simulink model "FLIGHT_Hexacopter_V2_1"  (R2024a)
settings: Solver=FixedStepDiscrete  StartTime=0.0  StopTime=inf  FixedStep=SampleTime_SAS  RelTol=1e-3  EnableMultiTasking=on
InitFcn:
  | Init_FLIGHT_Hexacopter
values from neighbouring files (symbols this model uses):
  d2r = pi/180    (= 0.0174532925199)    [Init_FLIGHT_Hexacopter.m]
  Jxx = 0.0211    [Init_FLIGHT_Hexacopter.m]
  Jyy = 0.0219    [Init_FLIGHT_Hexacopter.m]
  Jzz = 0.0366    [Init_FLIGHT_Hexacopter.m]
  Kpp = 3.3894    [Init_FLIGHT_Hexacopter_fromNCMS.m]
  Kpr = 3.3894    [Init_FLIGHT_Hexacopter_fromNCMS.m]
  MAX_CONTROL_ANGLE_PITCH = 30*pi/180    (= 0.523598775598)    [Init_FLIGHT_Hexacopter.m]    (also in Init_FLIGHT_Hexacopter_fromNCMS.m = 0.349065850399)
  MAX_CONTROL_ANGLE_RATE_PITCH = 360*pi/180    (= 6.28318530718)    [Init_FLIGHT_Hexacopter.m]    (also in Init_FLIGHT_Hexacopter_fromNCMS.m)
  MAX_CONTROL_ANGLE_RATE_ROLL = 360*pi/180    (= 6.28318530718)    [Init_FLIGHT_Hexacopter.m]    (also in Init_FLIGHT_Hexacopter_fromNCMS.m)
  MAX_CONTROL_ANGLE_RATE_Y = 120*pi/180    (= 2.09439510239)    [Init_FLIGHT_Hexacopter.m]    (also in Init_FLIGHT_Hexacopter_fromNCMS.m)
  MAX_CONTROL_ANGLE_ROLL = 30*pi/180    (= 0.523598775598)    [Init_FLIGHT_Hexacopter.m]    (also in Init_FLIGHT_Hexacopter_fromNCMS.m = 0.349065850399)
  MAX_CONTROL_VELOCITY_XY = 1.5    [Init_FLIGHT_Hexacopter.m]    (also in Init_FLIGHT_Hexacopter_fromNCMS.m)
  MAX_CONTROL_VELOCITY_Z = 1    [Init_FLIGHT_Hexacopter.m]    (also in Init_FLIGHT_Hexacopter_fromNCMS.m)
  SampleTime = 1/250    (= 0.004)    [Init_FLIGHT_Hexacopter.m]    (also in Init_FLIGHT_Hexacopter_fromNCMS.m = 0.01)
  SampleTime_SAS = 1/1000    (= 0.001)    [Init_FLIGHT_Hexacopter.m]
undefined symbols (not defined in the file or in its folder): arguments, DiscIntNeverNeededParam, event_sequence, id, log_levels, MPC_Z_D, MPC_Z_I, MPC_Z_P, timestamp
libraries: px4lib x42, simulink x9, px4Utilslib x8, px4uORBlib x8, slpidlib x5, simulink_extras x2, sharedtransform x1, px4Sensorslib x1, matrix_library x1
(part 1 of 3)
settings Model: ExtModeTrigDuration=10  Creator=sslee  LastModifiedBy=sslee
settings SolverCC: AlgebraicLoopSolver=TrustRegion  PositivePriorityOrder=on  MaxZcPerStep=1
settings OptimizationCC: EnhancedBackFolding=on  PassReuseOutputArgsAs=Individual arguments  ZeroExternalMemoryAtStartup=off  ZeroInternalMemoryAtStartup=off  MaxStackSize=64  OptimizeBlockOrder=speed  DifferentSizesBufferReuse=on  OptimizationCustomize=off  EfficientTunableParamExpr=on
settings DebuggingCC: ParameterTunabilityLossMsg=error  UnconnectedInputMsg=warning  UnconnectedOutputMsg=warning  UnconnectedLineMsg=warning  SymbolicDimsDataTypeCodeGenerationDiagnostic=none
settings HardwareCC: ProdBitPerPointer=32  ProdBitPerSizeT=32  ProdBitPerPtrDiffT=32  ProdLargestAtomicInteger=Long  ProdLargestAtomicFloat=Double  ProdWordSize=32  ProdLongLongMode=on  ProdHWDeviceType=ARM Compatible->ARM Cortex
settings ModelReferenceCC: EnableRefExpFcnMdlSchedulingChecks=on
settings SFSimCC: MATLABDynamicMemAlloc=off  SimTargetLang=C++
settings RTWCC: Description=Embedded Coder  SystemTargetFile=ert.tlc  HardwareBoard=PX4 Pixhawk 6x  TLCOptions="-aInlineSetEventsForThisBaseRateFcn=TLC_FALSE -aSuppressMultiTaskScheduler=TLC_FALSE  -aRateBasedStepFcn=0"  TemplateMakefile=ert_default_tmf  Toolchain=GNU Tools for PX4 Autopilots  IncludeHyperlinkInReport=on  TargetLang=C++  GPUComputeCapability=3.5  DLArmComputeVersion=19.05
settings CodeAppCC: ForceParamTrailComments=on  IgnoreCustomStorageClasses=off  OperatorAnnotations=on  SimulinkDataObjDesc=on  SFDataObjDesc=on  InsertBlockDesc=on
settings ERTTargetCC: ExtModeTransport=3  ExtModeStaticAlloc=on  ExtModeStaticAllocSize=1024  ExtModeMexFile=ext_xcp  ExtModeIntrfLevel=Level2 - Open

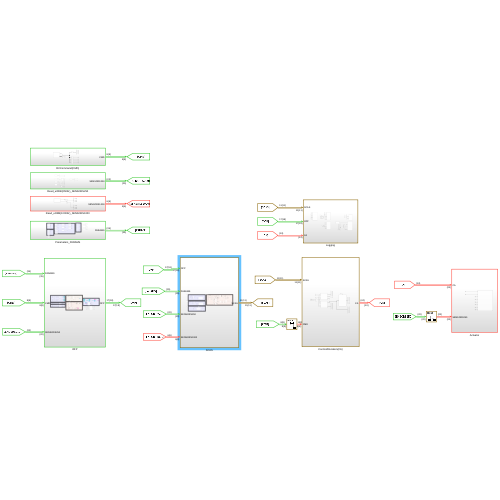
[thumbnail: Simulink's stored preview of the top-level diagram]
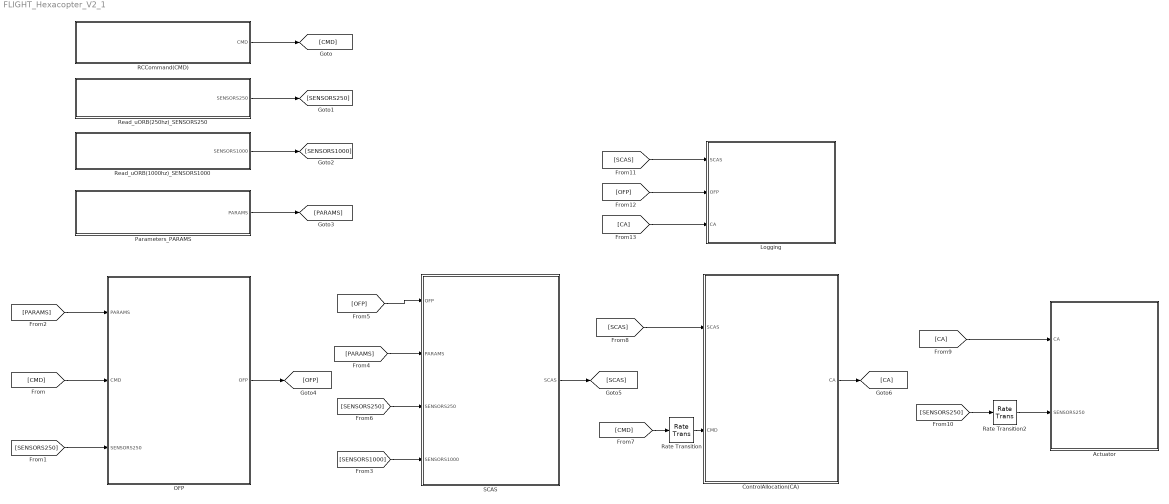
== system FLIGHT_Hexacopter_V2_1 ==
  Actuator : Subsystem
  ControlAllocation(CA) : Subsystem
  Logging : Subsystem
  OFP : Subsystem
  Parameters_PARAMS : Subsystem
  RCCommand(CMD) : Subsystem
  Rate Transition : RateTransition  OutPortSampleTime=SampleTime_SAS
  Rate Transition2 : RateTransition  OutPortSampleTime=SampleTime_SAS
  Read_uORB(1000hz)_SENSORS1000 : Subsystem
  Read_uORB(250hz)_SENSORS250 : Subsystem
  SCAS : Subsystem
  wires:
  [SENSORS250] -> OFP/3(SENSORS250)
  Read_uORB(1000hz)_SENSORS1000/1(SENSORS1000) -> [SENSORS1000]
  RCCommand(CMD)/1(CMD) -> [CMD]
  Read_uORB(250hz)_SENSORS250/1(SENSORS250) -> [SENSORS250]
  [CMD] -> OFP/2(CMD)
  Parameters_PARAMS/1(PARAMS) -> [PARAMS]
  [PARAMS] -> OFP/1(PARAMS)
  OFP/1(OFP) -> [OFP]
  [OFP] -> SCAS/1(OFP)
  [PARAMS] -> SCAS/2(PARAMS)
  [SENSORS250] -> SCAS/3(SENSORS250)
  [SENSORS1000] -> SCAS/4(SENSORS1000)
  [CMD] -> Rate Transition/1
  SCAS/1(SCAS) -> [SCAS]
  [SCAS] -> ControlAllocation(CA)/1(SCAS)
  Rate Transition/1 -> ControlAllocation(CA)/2(CMD)
  ControlAllocation(CA)/1(CA) -> [CA]
  [CA] -> Actuator/1(CA)
  [SENSORS250] -> Rate Transition2/1
  [SCAS] -> Logging/1(SCAS)
  [OFP] -> Logging/2(OFP)
  [CA] -> Logging/3(CA)
  Rate Transition2/1 -> Actuator/2(SENSORS250)

== system FLIGHT_Hexacopter_V2_1/Actuator ==
  BusElementIn : Inport  PortName=CA  Element=pwm_after_fault_m1
  BusElementIn1 : Inport  PortName=CA  Element=pwm_after_fault_m2
  BusElementIn2 : Inport  PortName=CA  Element=pwm_after_fault_m3
  BusElementIn3 : Inport  PortName=CA  Element=pwm_after_fault_m4
  BusElementIn4 : Inport  PortName=CA  Element=pwm_after_fault_m5
  BusElementIn5 : Inport  PortName=CA  Element=pwm_after_fault_m6
  BusElementIn6 : Inport  Port=2  PortName=SENSORS250  Element=VehicleStatus_flag_armed
  BusElementIn7 : Inport  Port=2  PortName=SENSORS250  Element=VehicleStatus_flag_kill
  PX4 PWM Output : px4lib/PX4 PWM Output  pwmDevice=Main  pwmChannel1_=on  pwmChannel2_=on  pwmChannel3_=on  pwmChannel4_=on  pwmChannel5_=on  pwmChannel6_=on  pwmChannel7_=off  pwmChannel8_=off
      settings: SourceProductName=UAV Toolbox Support Package for PX4 Autopilots
  wires:
  BusElementIn/1 -> PX4 PWM Output/3
  BusElementIn1/1 -> PX4 PWM Output/4
  BusElementIn2/1 -> PX4 PWM Output/5
  BusElementIn3/1 -> PX4 PWM Output/6
  BusElementIn4/1 -> PX4 PWM Output/7
  BusElementIn5/1 -> PX4 PWM Output/8
  BusElementIn6/1 -> PX4 PWM Output/1
  BusElementIn7/1 -> PX4 PWM Output/2

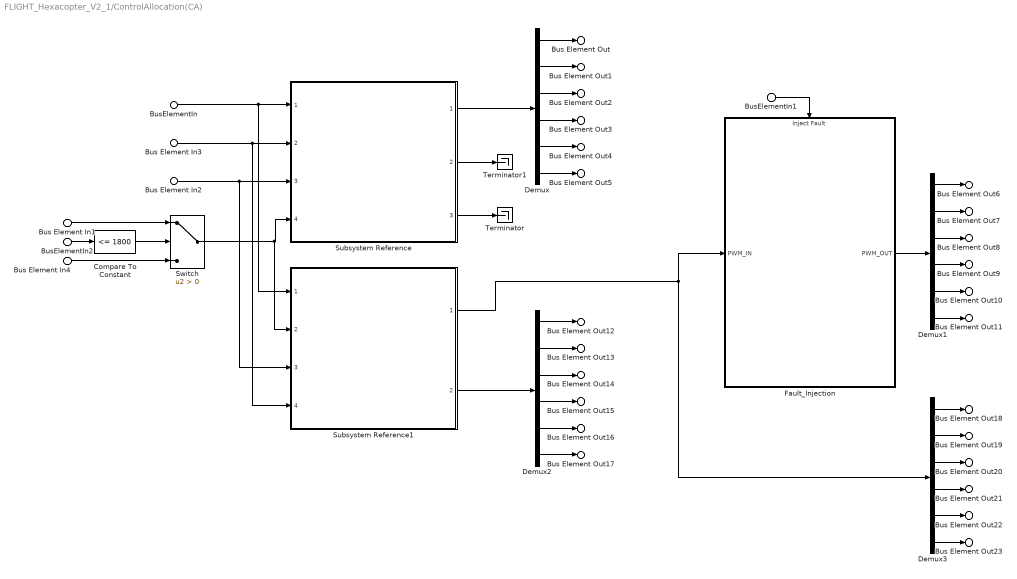
== system FLIGHT_Hexacopter_V2_1/ControlAllocation(CA) ==
  Bus Element In1 : Inport  PortName=SCAS  Element=tau_roll
  Bus Element In2 : Inport  PortName=SCAS  Element=tau_pitch
  Bus Element In3 : Inport  PortName=SCAS  Element=tau_yaw
  BusElementIn : Inport  PortName=SCAS  Element=tau_throttle
  Bus Element In4 : Inport  PortName=SCAS  Element=tau_roll_smc
  BusElementIn1 : Inport  Port=2  PortName=CMD  Element=rc_inject_failure
  BusElementIn2 : Inport  Port=2  PortName=CMD  Element=rc_ctrl_switch
  Compare To Constant : simulink/Logic and Bit Operations/Compare To Constant  relop=<=  const=1800  OutDataTypeStr=boolean
  Demux{,1..3} (4 alike) : Demux  Outputs=6
  Fault_Injection : Subsystem
      settings: PortSchema="{\"entries\":[{\"content\":{\"sides\":[{\"content\":{\"connectorIds\":[\"In1\"]},\"type\":\"ConnectorPlacement.EquallySpacedRectSide\",\"uuid\":\"fab26c65-8d77-46b7-b375-2033d08e8306\"},{\"content\":{\"connectorIds\":[\"Out1\"],\"side\":\"RIGHT\"},\"type\":\"ConnectorPlacement.EquallySpacedRectSide\",\"uuid\":\"bc3f50bd-e170-4b75-8089-4f92da68e83e\"},{\"content\":{\"connectorIds\":[\"In2\"],\"side\":\"TOP\"},\"type\":\"ConnectorPlacement.EquallySpacedRectSide\",\"uuid\":\"873ada90-6f93-48ab-a701-a52d28357753\"}]},\"type\":\"ConnectorPlacement.EquallySpacedConnector\",\"uuid\":\"201be8b3-bff4-4924-8e0c-28e5fee33d1c\"}],\"packageUris\":[\"http://schema.mathworks.com/mf0/Connector/R2020b\"],\"version\":\"1.0\"}"
  Subsystem Reference : Subsystem  ReferencedSubsystem=F550_ControlAllocation_sub_ver2023b
  Subsystem Reference1 : Subsystem  ReferencedSubsystem=F550_Adam_CA
  Switch : Switch  Criteria=u2 > Threshold  SaturateOnIntegerOverflow=off  InputSameDT=off
  Terminator : Terminator
  Terminator1 : Terminator
  Bus Element Out : Outport  PortName=CA  Element=thr_m1
  Bus Element Out1 : Outport  PortName=CA  Element=thr_m2
  Bus Element Out2 : Outport  PortName=CA  Element=thr_m3
  Bus Element Out3 : Outport  PortName=CA  Element=thr_m4
  Bus Element Out4 : Outport  PortName=CA  Element=thr_m5
  Bus Element Out5 : Outport  PortName=CA  Element=thr_m6
  Bus Element Out12 : Outport  PortName=CA  Element=thr_adam_m1
  Bus Element Out13 : Outport  PortName=CA  Element=thr_adam_m2
  Bus Element Out14 : Outport  PortName=CA  Element=thr_adam_m3
  Bus Element Out15 : Outport  PortName=CA  Element=thr_adam_m4
  Bus Element Out16 : Outport  PortName=CA  Element=thr_adam_m5
  Bus Element Out17 : Outport  PortName=CA  Element=thr_adam_m6
  Bus Element Out6 : Outport  PortName=CA  Element=pwm_after_fault_m1
  Bus Element Out7 : Outport  PortName=CA  Element=pwm_after_fault_m2
  Bus Element Out8 : Outport  PortName=CA  Element=pwm_after_fault_m3
  Bus Element Out9 : Outport  PortName=CA  Element=pwm_after_fault_m4
  Bus Element Out10 : Outport  PortName=CA  Element=pwm_after_fault_m5
  Bus Element Out11 : Outport  PortName=CA  Element=pwm_after_fault_m6
  Bus Element Out18 : Outport  PortName=CA  Element=pwm_before_fault_m1
  Bus Element Out19 : Outport  PortName=CA  Element=pwm_before_fault_m2
  Bus Element Out20 : Outport  PortName=CA  Element=pwm_before_fault_m3
  Bus Element Out21 : Outport  PortName=CA  Element=pwm_before_fault_m4
  Bus Element Out22 : Outport  PortName=CA  Element=pwm_before_fault_m5
  Bus Element Out23 : Outport  PortName=CA  Element=pwm_before_fault_m6
  wires:
  BusElementIn/1 -> Subsystem Reference1/1, Subsystem Reference/1
  Bus Element In3/1 -> Subsystem Reference1/4, Subsystem Reference/2
  Bus Element In2/1 -> Subsystem Reference1/3, Subsystem Reference/3
  Subsystem Reference/1 -> Demux/1
  Demux/1 -> Bus Element Out/1
  Demux/2 -> Bus Element Out1/1
  Demux/3 -> Bus Element Out2/1
  Demux/4 -> Bus Element Out3/1
  Demux/5 -> Bus Element Out4/1
  Demux/6 -> Bus Element Out5/1
  Subsystem Reference1/2 -> Demux2/1
  Subsystem Reference1/1 -> Fault_Injection/1(PWM_IN), Demux3/1
  Demux2/1 -> Bus Element Out12/1
  Demux2/2 -> Bus Element Out13/1
  Demux2/3 -> Bus Element Out14/1
  Demux2/4 -> Bus Element Out15/1
  Demux2/5 -> Bus Element Out16/1
  Demux2/6 -> Bus Element Out17/1
  Subsystem Reference/2 -> Terminator1/1
  BusElementIn1/1 -> Fault_Injection/2(Inject Fault)
  Fault_Injection/1(PWM_OUT) -> Demux1/1
  Subsystem Reference/3 -> Terminator/1
  Demux1/1 -> Bus Element Out6/1
  Demux1/2 -> Bus Element Out7/1
  Demux1/3 -> Bus Element Out8/1
  Demux1/4 -> Bus Element Out9/1
  Demux1/5 -> Bus Element Out10/1
  Demux1/6 -> Bus Element Out11/1
  Demux3/1 -> Bus Element Out18/1
  Demux3/2 -> Bus Element Out19/1
  Demux3/3 -> Bus Element Out20/1
  Demux3/4 -> Bus Element Out21/1
  Demux3/5 -> Bus Element Out22/1
  Demux3/6 -> Bus Element Out23/1
  BusElementIn2/1 -> Compare To Constant/1
  Compare To Constant/1 -> Switch/2
  Bus Element In1/1 -> Switch/1
  Bus Element In4/1 -> Switch/3
  Switch/1 -> Subsystem Reference1/2, Subsystem Reference/4

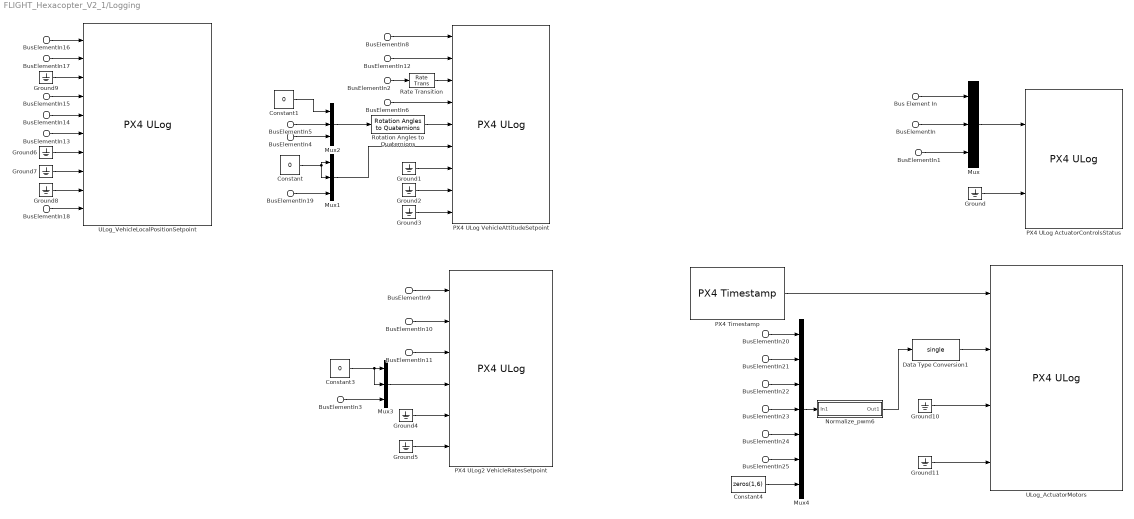
== system FLIGHT_Hexacopter_V2_1/Logging ==
  BusElementIn : Inport  PortName=SCAS  Element=tau_pitch
  BusElementIn1 : Inport  PortName=SCAS  Element=tau_yaw
  BusElementIn2 : Inport  PortName=SCAS  Element=tau_roll_smc
  BusElementIn4 : Inport  PortName=SCAS  Element=des_roll
  BusElementIn8 : Inport  PortName=SCAS  Element=des_roll
  BusElementIn5 : Inport  PortName=SCAS  Element=des_pitch
  BusElementIn6 : Inport  PortName=SCAS  Element=des_yr
  BusElementIn11 : Inport  PortName=SCAS  Element=des_yr
  BusElementIn9 : Inport  PortName=SCAS  Element=des_rollrate
  BusElementIn10 : Inport  PortName=SCAS  Element=des_pitchrate
  BusElementIn12 : Inport  PortName=SCAS  Element=smc_s
  Bus Element In : Inport  PortName=SCAS  Element=tau_roll
  BusElementIn13 : Inport  Port=2  PortName=OFP  Element=ATL_des_vz
  BusElementIn14 : Inport  Port=2  PortName=OFP  Element=POS_des_vy
  BusElementIn15 : Inport  Port=2  PortName=OFP  Element=POS_des_vx
  BusElementIn16 : Inport  Port=2  PortName=OFP  Element=POS_des_x
  BusElementIn17 : Inport  Port=2  PortName=OFP  Element=POS_des_y
  BusElementIn18 : Inport  Port=2  PortName=OFP  Element=des_yr
  BusElementIn19 : Inport  Port=2  PortName=OFP  Element=des_thr
  BusElementIn3 : Inport  Port=2  PortName=OFP  Element=des_thr
  BusElementIn20 : Inport  Port=3  PortName=CA  Element=pwm_after_fault_m1
  BusElementIn21 : Inport  Port=3  PortName=CA  Element=pwm_after_fault_m2
  BusElementIn22 : Inport  Port=3  PortName=CA  Element=pwm_after_fault_m3
  BusElementIn23 : Inport  Port=3  PortName=CA  Element=pwm_after_fault_m4
  BusElementIn24 : Inport  Port=3  PortName=CA  Element=pwm_after_fault_m5
  BusElementIn25 : Inport  Port=3  PortName=CA  Element=pwm_after_fault_m6
  Constant : Constant  Value=0  OutDataTypeStr=single
  Constant1 : Constant  Value=0  OutDataTypeStr=single  SampleTime=SampleTime
  Constant3 : Constant  Value=0  OutDataTypeStr=single
  Constant4 : Constant  Value=zeros(1,6)  OutDataTypeStr=uint16  SampleTime=SampleTime_SAS
  Data Type Conversion1 : DataTypeConversion  OutDataTypeStr=single  SaturateOnIntegerOverflow=off  RndMeth=Floor
  Ground{,1..11} (12 alike) : Ground
  Mux{,1..3} (4 alike) : Mux  Inputs=3
  Mux4 : Mux  Inputs=7
  Normalize_pwm6 : Subsystem
  PX4 Timestamp : px4Utilslib/PX4 Timestamp  SampleTime=SampleTime_SAS
      settings: SourceProductName=PX4 Utility Blocks
  PX4 ULog ActuatorControlsStatus : px4Utilslib/PX4 ULog  uORBTopic=ActuatorControlsStatus
      settings: SourceProductName=PX4 Utility Blocks
  PX4 ULog VehicleAttitudeSetpoint : px4Utilslib/PX4 ULog  uORBTopic=VehicleAttitudeSetpoint
      settings: SourceProductName=PX4 Utility Blocks
  PX4 ULog2 VehicleRatesSetpoint : px4Utilslib/PX4 ULog  uORBTopic=VehicleRatesSetpoint
      settings: SourceProductName=PX4 Utility Blocks
  Rate Transition : RateTransition  OutPortSampleTime=SampleTime
  Rotation Angles to Quaternions : sharedtransform/Rotation Angles to Quaternions  rotationOrder=ZYX  aMode=aMode
  ULog_ActuatorMotors : px4Utilslib/PX4 ULog  uORBTopic=ActuatorMotors
      settings: SourceProductName=PX4 Utility Blocks
  ULog_VehicleLocalPositionSetpoint : px4Utilslib/PX4 ULog  uORBTopic=VehicleLocalPositionSetpoint
      settings: SourceProductName=PX4 Utility Blocks
  wires:
  BusElementIn1/1 -> Mux/3
  Bus Element In/1 -> Mux/1
  BusElementIn/1 -> Mux/2
  BusElementIn4/1 -> Mux2/3
  Constant1/1 -> Mux2/1
  Mux2/1 -> Rotation Angles to Quaternions/1
  BusElementIn5/1 -> Mux2/2
  Constant/1 -> Mux1/1, Mux1/2
  BusElementIn19/1 -> Mux1/3
  BusElementIn3/1 -> Mux3/3
  Constant3/1 -> Mux3/2, Mux3/1
  BusElementIn20/1 -> Mux4/1
  BusElementIn22/1 -> Mux4/3
  BusElementIn23/1 -> Mux4/4
  Normalize_pwm6/1(Out1) -> Data Type Conversion1/1
  Constant4/1 -> Mux4/7
  BusElementIn21/1 -> Mux4/2
  BusElementIn24/1 -> Mux4/5
  BusElementIn25/1 -> Mux4/6
  Mux4/1 -> Normalize_pwm6/1(In1)
  Data Type Conversion1/1 -> ULog_ActuatorMotors/2
  PX4 Timestamp/1 -> ULog_ActuatorMotors/1
  Ground10/1 -> ULog_ActuatorMotors/3
  Ground11/1 -> ULog_ActuatorMotors/4
  Mux/1 -> PX4 ULog ActuatorControlsStatus/1
  Ground/1 -> PX4 ULog ActuatorControlsStatus/2
  BusElementIn8/1 -> PX4 ULog VehicleAttitudeSetpoint/1
  BusElementIn12/1 -> PX4 ULog VehicleAttitudeSetpoint/2
  BusElementIn6/1 -> PX4 ULog VehicleAttitudeSetpoint/4
  Rotation Angles to Quaternions/1 -> PX4 ULog VehicleAttitudeSetpoint/5
  Ground1/1 -> PX4 ULog VehicleAttitudeSetpoint/7
  Ground2/1 -> PX4 ULog VehicleAttitudeSetpoint/8
  Ground3/1 -> PX4 ULog VehicleAttitudeSetpoint/9
  Mux1/1 -> PX4 ULog VehicleAttitudeSetpoint/6
  BusElementIn16/1 -> ULog_VehicleLocalPositionSetpoint/1
  BusElementIn17/1 -> ULog_VehicleLocalPositionSetpoint/2
  BusElementIn15/1 -> ULog_VehicleLocalPositionSetpoint/4
  BusElementIn14/1 -> ULog_VehicleLocalPositionSetpoint/5
  BusElementIn13/1 -> ULog_VehicleLocalPositionSetpoint/6
  Ground6/1 -> ULog_VehicleLocalPositionSetpoint/7
  Ground7/1 -> ULog_VehicleLocalPositionSetpoint/8
  Ground8/1 -> ULog_VehicleLocalPositionSetpoint/9
  BusElementIn18/1 -> ULog_VehicleLocalPositionSetpoint/10
  BusElementIn10/1 -> PX4 ULog2 VehicleRatesSetpoint/2
  BusElementIn11/1 -> PX4 ULog2 VehicleRatesSetpoint/3
  BusElementIn9/1 -> PX4 ULog2 VehicleRatesSetpoint/1
  Mux3/1 -> PX4 ULog2 VehicleRatesSetpoint/4
  Ground4/1 -> PX4 ULog2 VehicleRatesSetpoint/5
  Ground5/1 -> PX4 ULog2 VehicleRatesSetpoint/6
  Rate Transition/1 -> PX4 ULog VehicleAttitudeSetpoint/3
  BusElementIn2/1 -> Rate Transition/1
  Ground9/1 -> ULog_VehicleLocalPositionSetpoint/3

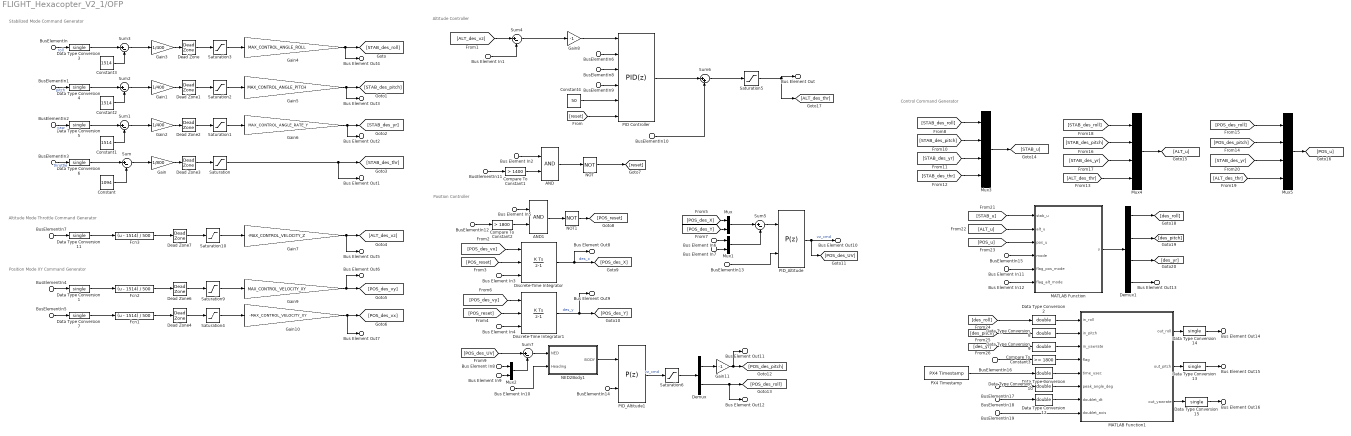
== system FLIGHT_Hexacopter_V2_1/OFP ==
  note: Control Command Generator
  note: Position Controller
  note: Altitude Controller
  note: Position Mode XY Command Generator
  note: Altitude Mode Throttle Command Generator
  note: Stabilized Mode Command Generator
  BusElementIn6 : Inport  PortName=PARAMS  Element=MPC_Z_VEL_P_ACC
  BusElementIn8 : Inport  PortName=PARAMS  Element=MPC_Z_VEL_I_ACC
  BusElementIn9 : Inport  PortName=PARAMS  Element=MPC_Z_VEL_D_ACC
  BusElementIn10 : Inport  PortName=PARAMS  Element=MPC_THR_HOVER
  BusElementIn13 : Inport  PortName=PARAMS  Element=MPC_XY_P
  BusElementIn14 : Inport  PortName=PARAMS  Element=MPC_XY_VEL_P_ACC
  BusElementIn17 : Inport  PortName=PARAMS  Element=DOUBLET_PEAK_ANG
  BusElementIn18 : Inport  PortName=PARAMS  Element=DOUBLET_DT
  BusElementIn19 : Inport  PortName=PARAMS  Element=DOUBLET_AXIS
  BusElementIn : Inport  Port=2  PortName=CMD  Element=rc_roll
  BusElementIn4 : Inport  Port=2  PortName=CMD  Element=rc_roll
  BusElementIn1 : Inport  Port=2  PortName=CMD  Element=rc_pitch
  BusElementIn5 : Inport  Port=2  PortName=CMD  Element=rc_pitch
  BusElementIn2 : Inport  Port=2  PortName=CMD  Element=rc_yaw
  BusElementIn3 : Inport  Port=2  PortName=CMD  Element=rc_throttle
  BusElementIn7 : Inport  Port=2  PortName=CMD  Element=rc_throttle
  BusElementIn11 : Inport  Port=2  PortName=CMD  Element=rc_mode
  BusElementIn12 : Inport  Port=2  PortName=CMD  Element=rc_mode
  BusElementIn15 : Inport  Port=2  PortName=CMD  Element=rc_mode
  BusElementIn16 : Inport  Port=2  PortName=CMD  Element=rc_doublet
  Bus Element In1 : Inport  Port=3  PortName=SENSORS250  Element=W
  Bus Element In2 : Inport  Port=3  PortName=SENSORS250  Element=VehicleStatus_armed
  Bus Element In5 : Inport  Port=3  PortName=SENSORS250  Element=VehicleStatus_armed
  Bus Element In3 : Inport  Port=3  PortName=SENSORS250  Element=X
  Bus Element In6 : Inport  Port=3  PortName=SENSORS250  Element=X
  Bus Element In4 : Inport  Port=3  PortName=SENSORS250  Element=Y
  Bus Element In7 : Inport  Port=3  PortName=SENSORS250  Element=Y
  Bus Element In8 : Inport  Port=3  PortName=SENSORS250  Element=U
  Bus Element In9 : Inport  Port=3  PortName=SENSORS250  Element=V
  Bus Element In10 : Inport  Port=3  PortName=SENSORS250  Element=Heading
  Bus Element In11 : Inport  Port=3  PortName=SENSORS250  Element=VehicleStatus_flag_position_mode
  Bus Element In12 : Inport  Port=3  PortName=SENSORS250  Element=VehicleStatus_flag_altitude_mode
  AND : Logic  AllPortsSameDT=off  OutDataTypeStr=boolean
  AND1 : Logic  AllPortsSameDT=off  OutDataTypeStr=boolean
  Compare To Constant1 : simulink/Logic and Bit Operations/Compare To Constant  relop=>  const=1400  OutDataTypeStr=boolean
  Compare To Constant2 : simulink/Logic and Bit Operations/Compare To Constant  relop=>  const=1800  OutDataTypeStr=boolean
  Compare To Constant3 : simulink/Logic and Bit Operations/Compare To Constant  relop=>=  const=1800  OutDataTypeStr=boolean
  Constant : Constant  Value=1094
  Constant1 : Constant  Value=1514  OutDataTypeStr=single
  Constant2 : Constant  Value=1514  OutDataTypeStr=single
  Constant3 : Constant  Value=1514  OutDataTypeStr=single
  Constant4 : Constant  Value=50  OutDataTypeStr=single  SampleTime=SampleTime
  Data Type Conversion{,2,8..10,12} (6 alike) : DataTypeConversion  OutDataTypeStr=double  SaturateOnIntegerOverflow=off  RndMeth=Floor
  Data Type Conversion{1,3..7,11,13..15} (10 alike) : DataTypeConversion  OutDataTypeStr=single  SaturateOnIntegerOverflow=off  RndMeth=Floor
  Dead Zone : DeadZone  LowerValue=-0.005  UpperValue=0.005
  Dead Zone1 : DeadZone  LowerValue=-0.005  UpperValue=0.005
  Dead Zone2 : DeadZone  LowerValue=-0.005  UpperValue=0.005
  Dead Zone3 : DeadZone  LowerValue=-0.05  UpperValue=0.05
  Dead Zone4 : DeadZone  LowerValue=-0.1  UpperValue=0.1
  Dead Zone6 : DeadZone  LowerValue=-0.1  UpperValue=0.1
  Dead Zone7 : DeadZone  LowerValue=-0.1  UpperValue=0.1
  Demux : Demux  Outputs=2
  Demux1 : Demux
  Discrete-Time Integrator : DiscreteIntegrator  ExternalReset=level  InitialConditionSource=external  InitialCondition=SampleTime  SampleTime=SampleTime  LimitOutput=on  UpperSaturationLimit=+10  LowerSaturationLimit=-50  ICPrevOutput=DiscIntNeverNeededParam  ICPrevScaledInput=DiscIntNeverNeededParam
  Discrete-Time Integrator1 : DiscreteIntegrator  ExternalReset=level  InitialConditionSource=external  InitialCondition=SampleTime  SampleTime=SampleTime  LimitOutput=on  UpperSaturationLimit=+10  LowerSaturationLimit=-50  ICPrevOutput=DiscIntNeverNeededParam  ICPrevScaledInput=DiscIntNeverNeededParam
  Fcn1 : Fcn  Expr=(u - 1514) / 500
  Fcn2 : Fcn  Expr=(u - 1514) / 500
  Fcn3 : Fcn  Expr=(u - 1514) / 500
  Gain : Gain  Gain=1/800  OutDataTypeStr=single
  Gain1 : Gain  Gain=1/400  OutDataTypeStr=single
  Gain10 : Gain  Gain=-MAX_CONTROL_VELOCITY_XY
  Gain11 : Gain  Gain=-1
  Gain2 : Gain  Gain=1/400  OutDataTypeStr=single
  Gain3 : Gain  Gain=1/400  OutDataTypeStr=single
  Gain4 : Gain  Gain=MAX_CONTROL_ANGLE_ROLL
  Gain5 : Gain  Gain=MAX_CONTROL_ANGLE_PITCH
  Gain6 : Gain  Gain=MAX_CONTROL_ANGLE_RATE_Y
  Gain7 : Gain  Gain=-MAX_CONTROL_VELOCITY_Z
  Gain8 : Gain  Gain=-1
  Gain9 : Gain  Gain=MAX_CONTROL_VELOCITY_XY
  MATLAB Function : MATLAB Function  TreatAsAtomicUnit=on
  MATLAB Function1 : MATLAB Function  TreatAsAtomicUnit=on
  Mux : Mux  Inputs=2
  Mux1 : Mux  Inputs=2
  Mux2 : Mux  Inputs=2
  Mux3 : Mux
  Mux4 : Mux
  Mux5 : Mux
  NED2Body1 : Subsystem
  NOT : Logic  Operator=NOT  IconShape=distinctive  AllPortsSameDT=off  OutDataTypeStr=boolean
  NOT1 : Logic  Operator=NOT  IconShape=distinctive  AllPortsSameDT=off  OutDataTypeStr=boolean
  PID Controller : slpidlib/PID Controller  Controller=PID  Form=Parallel  TimeDomain=Discrete-time  UseExternalTs=off  SampleTime=SampleTime  IntegratorMethod=Forward Euler  FilterMethod=Forward Euler  ControllerParametersSource=external  P=1  I=1  UseKiTs=off  D=0  UseExternalDerivativeSource=off  N=100  UseFilter=on  TunerSelectOption=Transfer Function Based (PID Tuner App)  InitialConditionSource=internal  InitialConditionForIntegrator=0  InitialConditionForFilter=0  DifferentiatorICPrevScaledInput=0  ExternalReset=level  TrackingMode=off  Kt=1  LimitOutput=on  SatLimitsSource=internal  UpperSaturationLimit=1  LowerSaturationLimit=0  LinearizeAsGain=on  AntiWindupMode=clamping  Kb=1  LimitIntegrator=on  UpperIntegratorSaturationLimit=0.3  LowerIntegratorSaturationLimit=-0.3  POutMin=[]  POutMax=[]  IOutMin=[]  IOutMax=[]  DOutMin=[]  DOutMax=[]  NOutMin=[]  NOutMax=[]  SumOutMin=[]  SumOutMax=[]  SaturationOutMin=[]  SaturationOutMax=[]  PParamMin=[]  PParamMax=[]  IParamMin=[]  IParamMax=[]  DParamMin=[]  DParamMax=[]  NParamMin=[]  NParamMax=[]  KbParamMin=[]  KbParamMax=[]  KtParamMin=[]  KtParamMax=[]  KbOutMin=[]  KbOutMax=[]  KtOutMin=[]  KtOutMax=[]  IntegratorOutMin=[]  IntegratorOutMax=[]  FilterOutMin=[]  FilterOutMax=[]  SumI1OutMin=[]  SumI1OutMax=[]  SumI2OutMin=[]  SumI2OutMax=[]  SumI3OutMin=[]  SumI3OutMax=[]  SumI4OutMin=[]  SumI4OutMax=[]  SumDOutMin=[]  SumDOutMax=[]  DifferentiatorOutMin=[]  DifferentiatorOutMax=[]  FilterDiffOutCoefMin=[]  FilterDiffOutCoefMax=[]  ReciprocalOutMin=[]  ReciprocalOutMax=[]  SumDenOutMin=[]  SumDenOutMax=[]  SumNumOutMin=[]  SumNumOutMax=[]  DivideOutMin=[]  DivideOutMax=[]  UdiffTsProdOutMin=[]  UdiffTsProdOutMax=[]  NTsProdOutMin=[]  NTsProdOutMax=[]  UintegralTsProdOutMin=[]  UintegralTsProdOutMax=[]  UngainTsProdOutMin=[]  UngainTsProdOutMax=[]  ClampingZeroOutDataTypeStr=Inherit: Inherit via back propagation  ClampingZeroOutMin=[]  ClampingZeroOutMax=[]  FilterDenConstantOutDataTypeStr=Inherit: Inherit via back propagation  FilterDenConstantOutMin=[]  FilterDenConstantOutMax=[]  PCopyOutDataTypeStr=Inherit: Inherit via back propagation  PCopyOutMin=[]  PCopyOutMax=[]  NCopyOutDataTypeStr=Inherit: Inherit via back propagation  NCopyOutMin=[]  NCopyOutMax=[]  IntegratorContinuousStateAttributes=''  IntegratorStateMustResolveToSignalObject=off  IntegratorRTWStateStorageClass=Auto  FilterContinuousStateAttributes=''  FilterStateMustResolveToSignalObject=off  FilterRTWStateStorageClass=Auto  ParallelPVariant=ExternalParameters  IdealPVariant=Disabled  IVariant=ExternalParameters  DVariant=ExternalParameters  IntegratorVariant=Discrete  SatVariant=Enabled  AWVariant=DiscClampingParallel  PCopyVariant=Disabled  TRVariant=Disabled  FdbkBlocksVariant=Forward  IdealPFdbkVariant=Disabled  SatFdbkVariant=Disabled  DerivativeFilterVariant=ForwardEulerFilter  NVariant=ExternalParameters  NCopyVariant=Disabled  FilterICVariant=InternalICsFilter  IntegratorICVariant=InternalICs  ExternalResetVariant=ExternalReset  TRSumVariant=Passthrough  SumFdbkVariant=Disabled  SumVariant=Sum_PID  TsampFilterVariant=InternalTs  TsampNgainVariant=Passthrough  TsampIntegralVariant=Disabled_SignalSpec  ExternalSaturationOutDataTypeStr=Inherit: Same as second input  DerivativeSourceVariant=ErrorSignal
  PID_Altitude : slpidlib/PID Controller  Controller=P  Form=Parallel  TimeDomain=Discrete-time  UseExternalTs=off  SampleTime=-1  IntegratorMethod=Backward Euler  FilterMethod=Forward Euler  ControllerParametersSource=external  P=MPC_Z_P  I=MPC_Z_I  UseKiTs=off  D=MPC_Z_D  UseExternalDerivativeSource=off  N=10  UseFilter=on  TunerSelectOption=Transfer Function Based (PID Tuner App)  InitialConditionSource=internal  InitialConditionForIntegrator=0  InitialConditionForFilter=0  DifferentiatorICPrevScaledInput=0  ExternalReset=none  TrackingMode=off  Kt=1  LimitOutput=off  SatLimitsSource=internal  UpperSaturationLimit=inf  LowerSaturationLimit=-inf  LinearizeAsGain=off  AntiWindupMode=clamping  Kb=1  LimitIntegrator=off  UpperIntegratorSaturationLimit=inf  LowerIntegratorSaturationLimit=-inf  POutMin=[]  POutMax=[]  IOutMin=[]  IOutMax=[]  DOutMin=[]  DOutMax=[]  NOutMin=[]  NOutMax=[]  SumOutMin=[]  SumOutMax=[]  SaturationOutMin=[]  SaturationOutMax=[]  PParamMin=[]  PParamMax=[]  IParamMin=[]  IParamMax=[]  DParamMin=[]  DParamMax=[]  NParamMin=[]  NParamMax=[]  KbParamMin=[]  KbParamMax=[]  KtParamMin=[]  KtParamMax=[]  KbOutMin=[]  KbOutMax=[]  KtOutMin=[]  KtOutMax=[]  IntegratorOutMin=[]  IntegratorOutMax=[]  FilterOutMin=[]  FilterOutMax=[]  SumI1OutMin=[]  SumI1OutMax=[]  SumI2OutMin=[]  SumI2OutMax=[]  SumI3OutMin=[]  SumI3OutMax=[]  SumI4OutMin=[]  SumI4OutMax=[]  SumDOutMin=[]  SumDOutMax=[]  DifferentiatorOutMin=[]  DifferentiatorOutMax=[]  FilterDiffOutCoefMin=[]  FilterDiffOutCoefMax=[]  ReciprocalOutMin=[]  ReciprocalOutMax=[]  SumDenOutMin=[]  SumDenOutMax=[]  SumNumOutMin=[]  SumNumOutMax=[]  DivideOutMin=[]  DivideOutMax=[]  UdiffTsProdOutMin=[]  UdiffTsProdOutMax=[]  NTsProdOutMin=[]  NTsProdOutMax=[]  UintegralTsProdOutMin=[]  UintegralTsProdOutMax=[]  UngainTsProdOutMin=[]  UngainTsProdOutMax=[]  ClampingZeroOutDataTypeStr=Inherit: Inherit via back propagation  ClampingZeroOutMin=[]  ClampingZeroOutMax=[]  FilterDenConstantOutDataTypeStr=Inherit: Inherit via back propagation  FilterDenConstantOutMin=[]  FilterDenConstantOutMax=[]  PCopyOutDataTypeStr=Inherit: Inherit via back propagation  PCopyOutMin=[]  PCopyOutMax=[]  NCopyOutDataTypeStr=Inherit: Inherit via back propagation  NCopyOutMin=[]  NCopyOutMax=[]  IntegratorContinuousStateAttributes=''  IntegratorStateMustResolveToSignalObject=off  IntegratorRTWStateStorageClass=Auto  FilterContinuousStateAttributes=''  FilterStateMustResolveToSignalObject=off  FilterRTWStateStorageClass=Auto  ParallelPVariant=ExternalParameters  IdealPVariant=Disabled  IVariant=Disabled  DVariant=Disabled  IntegratorVariant=Disabled  SatVariant=Disabled  AWVariant=Disabled  PCopyVariant=Disabled  TRVariant=Disabled  FdbkBlocksVariant=Forward  IdealPFdbkVariant=Disabled  SatFdbkVariant=Disabled  DerivativeFilterVariant=Disabled  NVariant=Disabled  NCopyVariant=Disabled_SignalSpec  FilterICVariant=Disabled  IntegratorICVariant=Disabled  ExternalResetVariant=Disabled  TRSumVariant=Passthrough  SumFdbkVariant=Disabled  SumVariant=Passthrough_P  TsampFilterVariant=InternalTs  TsampNgainVariant=Passthrough  TsampIntegralVariant=Disabled_SignalSpec  ExternalSaturationOutDataTypeStr=Inherit: Same as second input  DerivativeSourceVariant=Disabled
  PID_Altitude1 : slpidlib/PID Controller  Controller=P  Form=Parallel  TimeDomain=Discrete-time  UseExternalTs=off  SampleTime=-1  IntegratorMethod=Backward Euler  FilterMethod=Forward Euler  ControllerParametersSource=external  P=MPC_Z_P  I=MPC_Z_I  UseKiTs=off  D=MPC_Z_D  UseExternalDerivativeSource=off  N=10  UseFilter=on  TunerSelectOption=Transfer Function Based (PID Tuner App)  InitialConditionSource=internal  InitialConditionForIntegrator=0  InitialConditionForFilter=0  DifferentiatorICPrevScaledInput=0  ExternalReset=none  TrackingMode=off  Kt=1  LimitOutput=off  SatLimitsSource=internal  UpperSaturationLimit=inf  LowerSaturationLimit=-inf  LinearizeAsGain=off  AntiWindupMode=clamping  Kb=1  LimitIntegrator=off  UpperIntegratorSaturationLimit=inf  LowerIntegratorSaturationLimit=-inf  POutMin=[]  POutMax=[]  IOutMin=[]  IOutMax=[]  DOutMin=[]  DOutMax=[]  NOutMin=[]  NOutMax=[]  SumOutMin=[]  SumOutMax=[]  SaturationOutMin=[]  SaturationOutMax=[]  PParamMin=[]  PParamMax=[]  IParamMin=[]  IParamMax=[]  DParamMin=[]  DParamMax=[]  NParamMin=[]  NParamMax=[]  KbParamMin=[]  KbParamMax=[]  KtParamMin=[]  KtParamMax=[]  KbOutMin=[]  KbOutMax=[]  KtOutMin=[]  KtOutMax=[]  IntegratorOutMin=[]  IntegratorOutMax=[]  FilterOutMin=[]  FilterOutMax=[]  SumI1OutMin=[]  SumI1OutMax=[]  SumI2OutMin=[]  SumI2OutMax=[]  SumI3OutMin=[]  SumI3OutMax=[]  SumI4OutMin=[]  SumI4OutMax=[]  SumDOutMin=[]  SumDOutMax=[]  DifferentiatorOutMin=[]  DifferentiatorOutMax=[]  FilterDiffOutCoefMin=[]  FilterDiffOutCoefMax=[]  ReciprocalOutMin=[]  ReciprocalOutMax=[]  SumDenOutMin=[]  SumDenOutMax=[]  SumNumOutMin=[]  SumNumOutMax=[]  DivideOutMin=[]  DivideOutMax=[]  UdiffTsProdOutMin=[]  UdiffTsProdOutMax=[]  NTsProdOutMin=[]  NTsProdOutMax=[]  UintegralTsProdOutMin=[]  UintegralTsProdOutMax=[]  UngainTsProdOutMin=[]  UngainTsProdOutMax=[]  ClampingZeroOutDataTypeStr=Inherit: Inherit via back propagation  ClampingZeroOutMin=[]  ClampingZeroOutMax=[]  FilterDenConstantOutDataTypeStr=Inherit: Inherit via back propagation  FilterDenConstantOutMin=[]  FilterDenConstantOutMax=[]  PCopyOutDataTypeStr=Inherit: Inherit via back propagation  PCopyOutMin=[]  PCopyOutMax=[]  NCopyOutDataTypeStr=Inherit: Inherit via back propagation  NCopyOutMin=[]  NCopyOutMax=[]  IntegratorContinuousStateAttributes=''  IntegratorStateMustResolveToSignalObject=off  IntegratorRTWStateStorageClass=Auto  FilterContinuousStateAttributes=''  FilterStateMustResolveToSignalObject=off  FilterRTWStateStorageClass=Auto  ParallelPVariant=ExternalParameters  IdealPVariant=Disabled  IVariant=Disabled  DVariant=Disabled  IntegratorVariant=Disabled  SatVariant=Disabled  AWVariant=Disabled  PCopyVariant=Disabled  TRVariant=Disabled  FdbkBlocksVariant=Forward  IdealPFdbkVariant=Disabled  SatFdbkVariant=Disabled  DerivativeFilterVariant=Disabled  NVariant=Disabled  NCopyVariant=Disabled_SignalSpec  FilterICVariant=Disabled  IntegratorICVariant=Disabled  ExternalResetVariant=Disabled  TRSumVariant=Passthrough  SumFdbkVariant=Disabled  SumVariant=Passthrough_P  TsampFilterVariant=InternalTs  TsampNgainVariant=Passthrough  TsampIntegralVariant=Disabled_SignalSpec  ExternalSaturationOutDataTypeStr=Inherit: Same as second input  DerivativeSourceVariant=Disabled
  PX4 Timestamp : px4Utilslib/PX4 Timestamp  SampleTime=SampleTime
      settings: SourceProductName=PX4 Utility Blocks
  Saturation : Saturate  UpperLimit=0.90  LowerLimit=0
  Saturation{1..4,9..10} (6 alike) : Saturate  UpperLimit=1  LowerLimit=-1
  Saturation5 : Saturate  UpperLimit=1  LowerLimit=0  OutDataTypeStr=single
  Saturation6 : Saturate  UpperLimit=35*d2r  LowerLimit=-35*d2r
  Sum{,1..5,7} (7 alike) : Sum  Inputs=|+-
  Sum6 : Sum  Inputs=|++  OutDataTypeStr=single
  Bus Element Out : Outport  PortName=OFP  Element=ALT_des_thr
  Bus Element Out1 : Outport  PortName=OFP  Element=STAB_des_thr
  Bus Element Out2 : Outport  PortName=OFP  Element=STAB_des_yr
  Bus Element Out3 : Outport  PortName=OFP  Element=STAB_des_pitch
  Bus Element Out4 : Outport  PortName=OFP  Element=STAB_des_roll
  Bus Element Out5 : Outport  PortName=OFP  Element=ATL_des_vz
  Bus Element Out6 : Outport  PortName=OFP  Element=POS_des_vy
  Bus Element Out7 : Outport  PortName=OFP  Element=POS_des_vx
  Bus Element Out8 : Outport  PortName=OFP  Element=POS_des_x
  Bus Element Out9 : Outport  PortName=OFP  Element=POS_des_y
  Bus Element Out10 : Outport  PortName=OFP  Element=POS_des_UV
  Bus Element Out11 : Outport  PortName=OFP  Element=POS_des_pitch
  Bus Element Out12 : Outport  PortName=OFP  Element=POS_des_roll
  Bus Element Out13 : Outport  PortName=OFP  Element=des_thr
  Bus Element Out14 : Outport  PortName=OFP  Element=des_roll
  Bus Element Out15 : Outport  PortName=OFP  Element=des_pitch
  Bus Element Out16 : Outport  PortName=OFP  Element=des_yr
  wires:
  Gain6/1 -> Bus Element Out2/1, [STAB_des_yr]
  Gain/1 -> Dead Zone3/1
  Sum2/1 -> Gain1/1
  BusElementIn3/1 -> Data Type Conversion6/1  "throttle"
  Saturation1/1 -> Gain6/1
  BusElementIn2/1 -> Data Type Conversion5/1  "yaw"
  Dead Zone/1 -> Saturation3/1
  Constant/1 -> Sum/2
  Constant3/1 -> Sum3/2
  BusElementIn/1 -> Data Type Conversion3/1  "roll"
  Constant2/1 -> Sum2/2
  Sum1/1 -> Gain2/1
  Sum/1 -> Gain/1
  Sum3/1 -> Gain3/1
  Dead Zone1/1 -> Saturation2/1
  BusElementIn1/1 -> Data Type Conversion4/1  "pitch"
  Dead Zone2/1 -> Saturation1/1
  Saturation2/1 -> Gain5/1
  Constant1/1 -> Sum1/2
  Gain1/1 -> Dead Zone1/1
  Gain2/1 -> Dead Zone2/1
  Dead Zone3/1 -> Saturation/1
  Saturation3/1 -> Gain4/1
  Gain3/1 -> Dead Zone/1
  Saturation/1 -> Bus Element Out1/1, [STAB_des_thr]
  Gain5/1 -> Bus Element Out3/1, [STAB_des_pitch]
  Gain4/1 -> Bus Element Out4/1, [STAB_des_roll]
  Dead Zone7/1 -> Saturation10/1
  Fcn3/1 -> Dead Zone7/1
  Data Type Conversion11/1 -> Fcn3/1
  Saturation10/1 -> Gain7/1
  Gain7/1 -> Bus Element Out5/1, [ALT_des_vz]
  BusElementIn7/1 -> Data Type Conversion11/1
  Data Type Conversion3/1 -> Sum3/1
  Data Type Conversion4/1 -> Sum2/1
  Data Type Conversion5/1 -> Sum1/1
  Data Type Conversion6/1 -> Sum/1
  Data Type Conversion7/1 -> Fcn1/1
  Fcn2/1 -> Dead Zone6/1
  Gain10/1 -> Bus Element Out7/1, [POS_des_vx]
  BusElementIn5/1 -> Data Type Conversion7/1
  Saturation9/1 -> Gain9/1
  Saturation4/1 -> Gain10/1
  Dead Zone6/1 -> Saturation9/1
  Data Type Conversion1/1 -> Fcn2/1
  Dead Zone4/1 -> Saturation4/1
  Fcn1/1 -> Dead Zone4/1
  BusElementIn4/1 -> Data Type Conversion1/1
  Gain9/1 -> Bus Element Out6/1, [POS_des_vy]
  Gain8/1 -> PID Controller/1
  [reset] -> PID Controller/6
  BusElementIn6/1 -> PID Controller/2
  Sum4/1 -> Gain8/1
  Bus Element In1/1 -> Sum4/2
  Sum6/1 -> Saturation5/1
  PID Controller/1 -> Sum6/1
  Constant4/1 -> PID Controller/5
  Saturation5/1 -> [ALT_des_thr], Bus Element Out/1
  [ALT_des_vz] -> Sum4/1
  BusElementIn8/1 -> PID Controller/3
  BusElementIn9/1 -> PID Controller/4
  BusElementIn10/1 -> Sum6/2
  BusElementIn11/1 -> Compare To Constant1/1
  Compare To Constant1/1 -> AND/2
  AND/1 -> NOT/1
  NOT/1 -> [reset]
  Bus Element In2/1 -> AND/1
  Discrete-Time Integrator/1 -> [POS_des_X], Bus Element Out8/1  "des_x"
  [POS_reset] -> Discrete-Time Integrator/2
  Discrete-Time Integrator1/1 -> [POS_des_Y], Bus Element Out9/1  "des_y"
  [POS_des_vx] -> Discrete-Time Integrator/1
  [POS_des_vy] -> Discrete-Time Integrator1/1
  [POS_reset] -> Discrete-Time Integrator1/2
  Bus Element In3/1 -> Discrete-Time Integrator/3
  Bus Element In4/1 -> Discrete-Time Integrator1/3
  Compare To Constant2/1 -> AND1/2
  NOT1/1 -> [POS_reset]
  BusElementIn12/1 -> Compare To Constant2/1
  Bus Element In5/1 -> AND1/1
  AND1/1 -> NOT1/1
  BusElementIn13/1 -> PID_Altitude/2
  Mux/1 -> Sum5/1
  PID_Altitude/1 -> [POS_des_UV], Bus Element Out10/1  "vz_cmd"
  Sum5/1 -> PID_Altitude/1
  [POS_des_X] -> Mux/1
  [POS_des_Y] -> Mux/2
  Bus Element In6/1 -> Mux1/1
  Bus Element In7/1 -> Mux1/2
  Mux1/1 -> Sum5/2
  Demux/2 -> Bus Element Out12/1, [POS_des_roll]
  Sum7/1 -> NED2Body1/1(NED)
  NED2Body1/1(BODY) -> PID_Altitude1/1
  Bus Element In10/1 -> NED2Body1/2(Heading)
  PID_Altitude1/1 -> Saturation6/1  "vz_cmd"
  Saturation6/1 -> Demux/1
  Gain11/1 -> Bus Element Out11/1, [POS_des_pitch]
  Demux/1 -> Gain11/1
  [POS_des_UV] -> Sum7/1
  Bus Element In8/1 -> Mux2/1
  Bus Element In9/1 -> Mux2/2
  Mux2/1 -> Sum7/2
  BusElementIn14/1 -> PID_Altitude1/2
  [STAB_des_roll] -> Mux3/1
  [STAB_des_pitch] -> Mux3/2
  [STAB_des_yr] -> Mux3/3
  [STAB_des_thr] -> Mux3/4
  Mux3/1 -> [STAB_u]
  [STAB_des_roll] -> Mux4/1
  [STAB_des_pitch] -> Mux4/2
  [STAB_des_yr] -> Mux4/3
  [ALT_des_thr] -> Mux4/4
  Mux4/1 -> [ALT_u]
  Mux5/1 -> [POS_u]
  [POS_des_roll] -> Mux5/1
  [POS_des_pitch] -> Mux5/2
  [STAB_des_yr] -> Mux5/3
  [ALT_des_thr] -> Mux5/4
  [STAB_u] -> MATLAB Function/1(stab_u)
  [ALT_u] -> MATLAB Function/2(alt_u)
  [POS_u] -> MATLAB Function/3(pos_u)
  BusElementIn15/1 -> MATLAB Function/4(mode)
  Bus Element In11/1 -> MATLAB Function/5(flag_pos_mode)
  Bus Element In12/1 -> MATLAB Function/6(flag_alt_mode)
  MATLAB Function/1(y) -> Demux1/1
  Demux1/1 -> [des_roll]
  Demux1/2 -> [des_pitch]
  Demux1/3 -> [des_yr]
  Demux1/4 -> Bus Element Out13/1
  Data Type Conversion13/1 -> Bus Element Out15/1
  Data Type Conversion9/1 -> MATLAB Function1/3(in_yawrate)
  Compare To Constant3/1 -> MATLAB Function1/4(flag)
  BusElementIn18/1 -> Data Type Conversion12/1
  MATLAB Function1/1(out_roll) -> Data Type Conversion14/1
  Data Type Conversion10/1 -> MATLAB Function1/6(peak_angle_deg)
  Data Type Conversion2/1 -> MATLAB Function1/1(in_roll)
  PX4 Timestamp/1 -> Data Type Conversion/1
  [des_pitch] -> Data Type Conversion8/1
  MATLAB Function1/3(out_yawrate) -> Data Type Conversion15/1
  BusElementIn16/1 -> Compare To Constant3/1
  Data Type Conversion12/1 -> MATLAB Function1/7(doublet_dt)
  BusElementIn19/1 -> MATLAB Function1/8(doublet_axis)
  [des_yr] -> Data Type Conversion9/1
  Data Type Conversion15/1 -> Bus Element Out16/1
  BusElementIn17/1 -> Data Type Conversion10/1
  Data Type Conversion/1 -> MATLAB Function1/5(time_usec)
  Data Type Conversion8/1 -> MATLAB Function1/2(in_pitch)
  MATLAB Function1/2(out_pitch) -> Data Type Conversion13/1
  [des_roll] -> Data Type Conversion2/1
  Data Type Conversion14/1 -> Bus Element Out14/1
